simulink model "IPAModell"  (R2020b)
settings: Solver=VariableStepAuto  StartTime=0.0  StopTime=10000  RelTol=1e-3
libraries: mcbcontrolslib x1, autolibpmsminterior x1
settings Model: EnablePacing=on  PacingRate=0.089000  Creator=unix  LastModifiedBy=unix

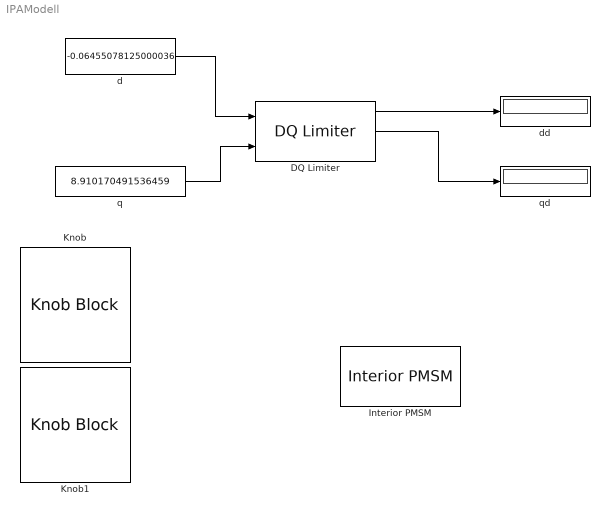
== system IPAModell ==
  DQ Limiter : mcbcontrolslib/DQ Limiter  Vmax=5.77
      settings: SourceProductBaseCode=MT
  Interior PMSM : autolibpmsminterior/Interior PMSM  port_config=Torque  sim_type=Discrete  Ts=2e-4  P=4  Rs=0.0449  Ldq=[1.117e-4 1.35e-4]  KConstText=Back-emf constant (Ke):  lambda_pm=0.2205  Ke=1.83  mechanical=[20.4e-6,4.924e-4,5e-3]  idq0=[0 0]  theta_init=0  omega_init=0  KConst=1.83  lambda_pm_calc=0.0025223  Kt=0.07  RefBlkName='autolibpmsminterior/Interior PMSM'  aMode=5
      settings: SourceProductBaseCode=PW,MT,UV,VE,VP
  Knob : KnobBlock  ScaleMin=-10  ScaleMax=10
  Knob1 : KnobBlock  ScaleMin=-10  ScaleMax=10
  d : Constant  Value=-0.06455078125000036  OutDataTypeStr=single
  dd : Display
  q : Constant  Value=8.910170491536459  OutDataTypeStr=single
  qd : Display
  wires:
  d/1 -> DQ Limiter/1
  q/1 -> DQ Limiter/2
  DQ Limiter/1 -> dd/1
  DQ Limiter/2 -> qd/1
